simulink model "Simulator"  (R2024b)
settings: Solver=FixedStepAuto  StartTime=0.0  StopTime=Parameters.Simulink.sim_time_s  FixedStep=Parameters.Simulink.time_step_s  RelTol=1e-6
undefined symbols (not defined in the file): att_0, data, flight_mode, FLIGHT_MODE, id, joystick, Parameters, res, timestamp, traj_opt, wait_time_s
libraries: dspsigops x3, simulink x2, eeGeneralControl x2, px4uORBlib x2, vrlib x1, simulink_extras x1, aerolibanimutils x1, sharedtransform x1
(part 2 of 2)

== system Simulator/Guidance/Subsystem2/minimum_snap/Subsystem/re-solve trajectory/Enabled Subsystem1/Subsystem3 ==
  States : Inport
  Bus Selector2 : BusSelector  OutputSignals=a_e,omega_dot
  Discrete Derivative : simulink/Discrete/Discrete Derivative  gainval=1.0  ICPrevScaledInput=0.0  OutMin=[]  OutMax=[]  OutDataType=fixdt(1, 16)  OutScaling=2^-10  DoSatur=off
  Discrete Derivative1 : simulink/Discrete/Discrete Derivative  gainval=1.0  ICPrevScaledInput=0.0  OutMin=[]  OutMax=[]  OutDataType=fixdt(1, 16)  OutScaling=2^-10  DoSatur=off
  Low-Pass Filter (Discrete or Continuous) : eeGeneralControl/Low-Pass Filter (Discrete or Continuous)  K=1  T=0.1  B=inf  A=-inf  init_option=Inherited from block input  x0=0  Ts=-1
  Low-Pass Filter (Discrete or Continuous)1 : eeGeneralControl/Low-Pass Filter (Discrete or Continuous)  K=1  T=0.1  B=inf  A=-inf  init_option=Inherited from block input  x0=0  Ts=-1
  Mux : Mux  Inputs=2
  Reshape : Reshape
  Reshape1 : Reshape
  Selector : Selector  InputPortWidth=3  IndexOptions=Index vector (dialog)  Indices=[3]  OutputSizes=1
  state_vec_jerk : Outport
  state_vec_snap : Outport  Port=2
  wires:
  Bus Selector2/1 -> Reshape/1  "<a_e>"
  Reshape1/1 -> Mux/2
  Selector/1 -> Reshape1/1
  Bus Selector2/2 -> Selector/1  "<omega_dot>"
  Reshape/1 -> Mux/1
  States/1 -> Bus Selector2/1
  Mux/1 -> Discrete Derivative/1
  Discrete Derivative/1 -> Low-Pass Filter (Discrete or Continuous)/1
  Low-Pass Filter (Discrete or Continuous)/1 -> Discrete Derivative1/1, state_vec_jerk/1
  Discrete Derivative1/1 -> Low-Pass Filter (Discrete or Continuous)1/1
  Low-Pass Filter (Discrete or Continuous)1/1 -> state_vec_snap/1

== system Simulator/Inbound Data/Subsystem4/Subsystem/Subsystem1/Sliders/Subsystem2/If Action Subsystem ==
  Action Port : ActionPort
  Clock : Clock
  Constant : Constant  Value=flight_mode.autonomous
  Constant1 : Constant  Value=flight_mode.position_hold
  Constant2 : Constant  Value=wait_time_s
  GreaterThan : RelationalOperator  Operator=<  OutDataTypeStr=boolean  RndMeth=Simplest  InputSameDT=off
  Multiport Switch1 : MultiPortSwitch  DataPortOrder=Zero-based contiguous  Inputs=2  DiagnosticForDefault=None  zeroidx=on  SaturateOnIntegerOverflow=off  InputSameDT=off
  Out1 : Outport
  wires:
  Constant2/1 -> GreaterThan/2
  Constant1/1 -> Multiport Switch1/3
  GreaterThan/1 -> Multiport Switch1/1
  Constant/1 -> Multiport Switch1/2
  Multiport Switch1/1 -> Out1/1
  Clock/1 -> GreaterThan/1

== system Simulator/Inbound Data/Subsystem4/Subsystem/Subsystem1/Sliders/Subsystem2/If Action Subsystem1 ==
  In1 : Inport
  Action Port : ActionPort
  Out1 : Outport
  wires:
  In1/1 -> Out1/1

== matlab function Simulator/Inbound Data/Subsystem3/Trajectory Solution/Call solver/Enabled Subsystem/MATLAB Function ==
  settings: updateMethod=DISCRETE  sampleTime=Parameters.Simulink.time_step_s
  data: trajectory_id input size=1; T_new output size=[1,100]; pp_new output size=[99,10,4]; n_dim_new output size=1; n_dim_ids_new output size=[4,1]; N_segments_new output size=1
function [T_new, pp_new, n_dim_new, n_dim_ids_new, N_segments_new]...
    = traj_solver(trajectory_id)
[wpts, Tf] = trajectory_manager.get_traj(trajectory_ID(trajectory_id));

opt_time_allocation_fl = false;
ShowDetails = false;

[T_new, pp_new, n_dim_new, n_dim_ids_new, N_segments_new, offset_new, Cost, ExitFlag, Iterations] = solver_codegen(wpts, Tf, ...
    opt_time_allocation_fl, ShowDetails);
end

== matlab function Simulator/Guidance/Subsystem2/minimum_snap/Subsystem/use static solution/MATLAB Function ==
  settings: updateMethod=DISCRETE  sampleTime=Parameters.Simulink.time_step_s
  data: t input size=1; p output size=[3,1]; v output size=[3,1]; a output size=[3,1]; jerk output size=[3,1]; T input double [0..]; coefs input double; snap output size=[3,1]; psi output size=1; psi_dot output size=1; psi_ddot output size=1; finished_traj output size=1; n_dim input; n_dim_src input; n_dim_ids input; n_int input; waypoints_offset input; gen_FF_fl input
function [p, v, a, jerk, snap, psi, psi_dot, psi_ddot, finished_traj] = eval_traj(...
    t,T,coefs,n_dim,n_dim_src, n_dim_ids, n_int, waypoints_offset, gen_FF_fl)

if isempty(T)
    finished_traj = true;
    p           = zeros(3,1);
    
    v           = zeros(3,1);
    p(:)        = waypoints_offset(1:3);
    a           = zeros(3,1);
    jerk        = zeros(3,1);
    snap        = zeros(3,1);
    psi         = waypoints_offset(4);
    psi_dot     = 0;
    psi_ddot    = 0;
else
    TU_input_factor = 10 / T(end);
    DU_input_factor = 1;
    
    if gen_FF_fl
        [p, v, a, jerk, snap, psi, psi_dot, psi_ddot, finished_traj] = eval_traj(...
            t,T,coefs,n_dim,n_dim_src, n_dim_ids, n_int, waypoints_offset, DU_input_factor, TU_input_factor);
    else
        [p, ~, ~, ~, ~, psi, ~, ~, finished_traj] = eval_traj(...
        t,T,coefs,n_dim,n_dim_src, n_dim_ids, n_int, waypoints_offset, DU_input_factor, TU_input_factor);
        v           = zeros(3,1);
        a           = zeros(3,1);
        jerk        = zeros(3,1);
        snap        = zeros(3,1);
        psi_dot     = 0;
        psi_ddot    = 0;
    end
end
end

== matlab function Simulator/Guidance/Subsystem2/Step input/MATLAB Function ==
  data: t input; pos output; yaw output; pos input; yaw input; completed output
function [pos, yaw, completed] = fcn(t, pos, yaw)
% pos = zeros(3,1);
% vel = zeros(3,1);
% att = zeros(3,1);
% att_rate = zeros(3,1);
completed = 0;

if t > 23
    completed = 1;
elseif t > 12
    pos(1) = pos(1) + 2;
    pos(2) = pos(2);
    pos(3) = pos(3) + 1;
elseif t > 6
    pos(1) = pos(1) + 2;
    pos(2) = pos(2);
else
    pos(1) = pos(1) + 1;
    pos(2) = pos(2) + 1;
end
end

== matlab function Simulator/Guidance/Subsystem2/minimum_snap/Subsystem/re-solve trajectory/Enabled Subsystem1/MATLAB Function ==
  settings: updateMethod=DISCRETE  sampleTime=Parameters.Simulink.time_step_s
  data: p output size=[3,1]; v output size=[3,1]; a output size=[3,1]; jerk output size=[3,1]; snap output size=[3,1]; psi output size=1; psi_dot output size=1; psi_ddot output size=1; finished_traj output size=1; guidance_active input; trajectory_id input size=1; time_since_start_of_traj_glob input size=1; update_dt input; T_glob input; pp_glob input; n_dim_glob input; n_dim_src_glob input; n_dim_ids_glob input; N_segments_glob input; state_0_glob input; time_since_start_of_traj output size=1; T output size=[1,100]; pp output size=[99,10,4]; n_dim output; n_dim_src output size=1; n_dim_ids output size=[4,1]; N_segments output size=1; state_0 output; state_vec input; detection_range input; waypoint_keepout_range input; collision_check_tol input; wpts output size=[4,100]
function [p, v, a, jerk, snap, psi, psi_dot, psi_ddot, finished_traj,...
            time_since_start_of_traj, T, pp, n_dim, n_dim_src, n_dim_ids, N_segments, state_0, wpts]...
            = update_and_eval_traj(guidance_active, trajectory_id, ...
            time_since_start_of_traj_glob, update_dt, ...
            T_glob, pp_glob, n_dim_glob, n_dim_src_glob, n_dim_ids_glob, N_segments_glob, ...
            state_0_glob, ...
            state_vec,... %, state_vec_vel, state_vec_acc, state_vec_jerk, state_vec_snap)
            detection_range, waypoint_keepout_range, collision_check_tol) 

persistent p_prev_ v_prev_ a_prev_ jerk_prev_ snap_prev_ psi_prev_ psi_dot_prev_ psi_ddot_prev_;

if (isempty(p_prev_) || isempty(v_prev_) || isempty(a_prev_) || isempty(jerk_prev_) || isempty(snap_prev_) || isempty(psi_prev_) ...
            || isempty(psi_dot_prev_) || isempty(psi_ddot_prev_))
    p_prev_ = zeros(3,1);
    p_prev_(:) = state_0_glob(1:3);
    v_prev_ = zeros(3,1);
    a_prev_ = zeros(3,1);
    jerk_prev_ = zeros(3,1);
    snap_prev_ = zeros(3,1);
    % psi_prev_ = 0;
    psi_prev_ = state_0_glob(4);
    psi_dot_prev_ = 0;
    psi_ddot_prev_ = 0;
end

[T, pp, n_dim, n_dim_src, n_dim_ids, N_segments, ...
    time_since_start_of_traj, state_0, wpts]...
            = traj_solver_...
            (guidance_active, trajectory_id, ...
            time_since_start_of_traj_glob, update_dt, ...
            T_glob, pp_glob, n_dim_glob, n_dim_src_glob, n_dim_ids_glob, N_segments_glob, ...
            state_0_glob, ...
            state_vec, ...% state_vec_vel, state_vec_acc, state_vec_jerk, state_vec_snap,...
            p_prev_, v_prev_, a_prev_, jerk_prev_, snap_prev_, psi_prev_, psi_dot_prev_, psi_ddot_prev_,...
            detection_range, waypoint_keepout_range, collision_check_tol);


[p, v, a, jerk, snap, psi, psi_dot, psi_ddot, finished_traj] = eval_traj_(...
    time_since_start_of_traj, T, pp, n_dim, n_dim_src, n_dim_ids, N_segments, state_0);


p_prev_(:) = p(1:3);
v_prev_(:) = v(1:3);
a_prev_(:) = a(1:3);
jerk_prev_(:) = jerk(1:3);
snap_prev_(:) = snap(1:3);
psi_prev_ = psi(1);
psi_dot_prev_ = psi_dot(1);
psi_ddot_prev_ = psi_ddot(1);

end


function [p, v, a, jerk, snap, psi, psi_dot, psi_ddot, finished_traj] = eval_traj_(...
    t,T,coefs,n_dim,n_dim_src, n_dim_ids, n_int, waypoints_offset)

    if isempty(T)
        finished_traj = true;
        p           = zeros(3,1);        
        v           = zeros(3,1);
        p(:)        = waypoints_offset(1:3);
        a           = zeros(3,1);
        jerk        = zeros(3,1);
        snap        = zeros(3,1);
        psi         = waypoints_offset(4);
        psi_dot     = 0;
        psi_ddot    = 0;
    else
        TU_input_factor = 10 / T(end);
        DU_input_factor = 1;
        
        [p, v, a, jerk, snap, psi, psi_dot, psi_ddot, finished_traj] = eval_traj(...
            t,T,coefs,n_dim,n_dim_src, n_dim_ids, n_int, waypoints_offset, DU_input_factor, TU_input_factor);
    end
end






function [T, pp, n_dim, n_dim_src, n_dim_ids, N_segments, ...
    time_since_start_of_traj, state_0, wpts]...
            = traj_solver_...
            (guidance_active, trajectory_id, ...
            time_since_start_of_traj_glob, update_dt, ...
            T_glob, pp_glob, n_dim_glob, n_dim_src_glob, n_dim_ids_glob, N_segments_glob, ...
            state_0_glob, ...
            state_vec, ...% state_vec_vel, state_vec_acc, state_vec_jerk, state_vec_snap,...
            p_prev, v_prev, a_prev, jerk_prev, snap_prev, psi_prev, psi_dot_prev, psi_ddot_prev,...
            detection_range, waypoint_keepout_range, collision_check_tol)
    
    %initialization:
    persistent T_  pp_ n_dim_ n_dim_src_ n_dim_ids_ N_segments_ time_since_start_of_traj_ status_int_ state_0_ wpts_ obstcl_;
    coder.varsize('T_',[1 inf], [0 1]);
    coder.varsize('pp_',[inf 10 inf]);
    coder.varsize('n_dim_ids_',[4 1], [1 0]);
    coder.varsize('wpts_',[4 inf], [1 1]);
    coder.varsize('obstcl_',[1 inf], [1 1]);
    
    if (isempty(obstcl_))
        [~, obstcl_] = trajectory_manager.get_traj(trajectory_ID(trajectory_id));
    end

    if (isempty(T_) || isempty(pp_) || isempty(n_dim_) || isempty(n_dim_src_) || isempty(n_dim_ids_) || isempty(N_segments_) ...
            || isempty(time_since_start_of_traj_) || isempty(status_int_) || isempty(state_0_)) || isempty(wpts_) ...
        T_ = T_glob(:)';
        pp_ = pp_glob;
        n_dim_ = n_dim_glob;
        n_dim_src_ = n_dim_src_glob;
        n_dim_ids_ = n_dim_ids_glob;
        N_segments_ = N_segments_glob;
        time_since_start_of_traj_ = time_since_start_of_traj_glob;
        status_int_ = 0;
        state_0_ = state_0_glob;
        [wpts_] = trajectory_manager.get_traj(trajectory_ID(trajectory_id));


        T = T_;
        pp = pp_;
        n_dim = n_dim_;
        n_dim_src = n_dim_src_;
        n_dim_ids = n_dim_ids_;
        N_segments = N_segments_;
        time_since_start_of_traj = time_since_start_of_traj_;
        state_0 = state_0_;
        wpts = wpts_;
        return;
    end

    % state_0 = zeros(4,1); %x, y, z, yaw

    if status_int_ == 2 && ~guidance_active
        status_int_ = 1;
    end

    switch status_int_
        case 2 % this time we will actually re-solve the trajectory            
            % the routine is after the switch-case 
            % (don't return here)

        case 1 % check timing and request to solve a trajectory (keep old result)
            % trajectory_update_dt_s = .1;

            % if rem(time_since_start_of_traj_glob,trajectory_update_dt_s) == 0 %time to update (time-based)
            for i = 1:length(obstcl_)
                if obstcl_{i}.check_if_obs_is_interior(state_vec(1:3), detection_range)
                    obstcl_{i}.is_visible = true;
                    if (~obstcl_{i}.was_processed)
                        if time_since_start_of_traj_glob > 0.0 && time_since_start_of_traj_ < T_(N_segments_+1)
                            disp(time_since_start_of_traj_glob)
                            status_int_ = 2;
                        end
                    end
                else
                    obstcl_{i}.is_visible = false;
                    % obstcl_{i}.was_processed = false;
                end
            end


            T = T_;
            pp = pp_;
            n_dim = n_dim_;
            n_dim_src = n_dim_src_;
            n_dim_ids = n_dim_ids_;
            N_segments = N_segments_;
            time_since_start_of_traj_ = (time_since_start_of_traj_ + update_dt);
            time_since_start_of_traj = time_since_start_of_traj_;
            state_0 = state_0_;
            wpts = wpts_;
            return;
            
            
        otherwise % don't solve anything just pass global solution and update status
            T_ = T_glob(:)';
            pp_ = pp_glob;
            n_dim_ = n_dim_glob;
            n_dim_src_ = n_dim_src_glob;
            n_dim_ids_ = n_dim_ids_glob;
            N_segments_ = N_segments_glob;
            time_since_start_of_traj_ = time_since_start_of_traj_glob;
            state_0_ = state_0_glob;
    
    
            T = T_;
            pp = pp_;
            n_dim = n_dim_;
            n_dim_src = n_dim_src_;
            n_dim_ids = n_dim_ids_;
            N_segments = N_segments_;
            time_since_start_of_traj = time_since_start_of_traj_;
            state_0 = state_0_;
            wpts = wpts_;
            
            if guidance_active && time_since_start_of_traj_glob > 0.0 && ~isempty(T_) && time_since_start_of_traj_glob < T_(N_segments_+1)
                %trajectory guidance is active, start checking stuff
                status_int_ = 1; 
            end
            return;
    end
    
    % use state:
    % state_0__ = state_vec(1:4); % we will output a new intial state
    
    % alternatively we can use the last setpoint:
    state_0__ = [p_prev(1:3); psi_prev(1)]; % we will output a new intial state

    %we want to remove the completed waypoints:
    completed_segments = time_since_start_of_traj_ + update_dt >= T_;
    N_remove_segments = nnz(completed_segments) - 1;

    N_segments_traj = size(wpts_,2) - 1;
    wpts_mod_ = wpts_(:,N_remove_segments+1:N_segments_traj+1); %for now, we make a local copy (we may discard this later)
    
    %let's evaluate the trajectory ahead of us to check for the collisions
    % first, we need to make sure we keep the "old" parameters needed for
    % trajectory evaluation (mainly time) 
    Tf =T_(N_segments_+1); % total flight time (for old trajectory)
    T_mod_ = T_(N_remove_segments+1:N_segments_traj+1) - time_since_start_of_traj_; %this is cropped time vector
    T_mod_(1) = 0; % make sure new time vector starts at 0
    eval_time_ahead__ = time_since_start_of_traj_+update_dt:0.1:T_(N_segments_+1); %evaluation has to be relative to the old time vector
    TU_input_factor__ = 10 / Tf; %time scaling (old)
    p_look_ahead__ = TrajectoryOptimizer.common.eval_pp(...
                eval_time_ahead__,...
                0,...
                pp_, ...
                T_, ...
                n_dim_,...
                n_dim_src_, ...
                n_dim_ids_, ...
                N_segments_, ...
                state_0_, ...
                1, ...
                TU_input_factor__); %we do this once and use to check all obstacles
    eval_time_ahead__ = eval_time_ahead__-time_since_start_of_traj_; %offset by the flown time 

    requires_trajectory_update = false; %we mat actually have no collision with any of the obstacles, so don't update just because... 
    
    for i = 1:length(obstcl_) %checking every obstacle
        if obstcl_{i}.is_visible && ~obstcl_{i}.was_processed %only visible and those that have not been processed yet
            [is_interior__, n_new_wpts__, new_wpts__, new_wpt_T__] = obstcl_{i}.check_traj(eval_time_ahead__, p_look_ahead__(1:3,:), collision_check_tol, waypoint_keepout_range);
            if nnz(is_interior__) > 0 % only if any of the points are inside the obstacles
                [wpts_mod_, T_mod_] = obstcl_{i}.insert_new_wpts(new_wpt_T__, n_new_wpts__, new_wpts__, wpts_mod_, T_mod_, collision_check_tol); %updates waypoints and time vector
                % obstcl_{i}.was_processed = true;
                requires_trajectory_update = true;
                for ii = 1:length(obstcl_)
                    if obstcl_{ii}.is_visible
                        obstcl_{ii}.was_processed = false;
                    end
                end
            end
        end
    end

    if requires_trajectory_update %only if needed
        %here we will compute a new trajectory based on the updated
        %waypoints and time vector
        T_ = T_mod_;
        wpts_ = wpts_mod_;
    
        Tf = T_(end);    
        wpts_(:,1) = state_0__(1:4);   
    
        opt_time_allocation_fl = false;
        ShowDetails = false;        
        timeWt = 0;
        
        scaling = 10;
        
        minSegmentTime = 0.1*diff(T_);
        maxSegmentTime = Tf;
        
        % wptFun = @(t) bcs_fun1__(t, wpts);
        wptFun = @(t) bcs_fun2__(t, wpts_, v_prev, a_prev, jerk_prev, snap_prev, psi_dot_prev, psi_ddot_prev);
        % wptFun = @(t)bcs_fun3__(t, wpts, state_vec_vel, state_vec_acc, state_vec_jerk, state_vec_snap);
        
        sol = TrajectoryOptimizer.solver_mexfriendy( ...
            T_,...
            opt_time_allocation_fl,...
            ShowDetails, ...
            wptFun, ...
            [], ...
            minSegmentTime, ...
            maxSegmentTime, ...
            timeWt, ...
            scaling / Tf);
        
        % stats = sol.get_stats;
        minsnap_set = sol.get_res;
    
        % ExitFlag = stats.ExitFlag;
        % Iterations = stats.Iterations;
        % Cost = stats.J;
    
        pp = minsnap_set.pp;
        T = minsnap_set.T;
        n_dim = minsnap_set.n_dim;
        n_dim_src = minsnap_set.n_dim_src;
        n_dim_ids = minsnap_set.n_dim_ids;
        N_segments = minsnap_set.N_segments;
        state_0 = state_0__;
        time_since_start_of_traj = update_dt;
    
        status_int_ = 1; %return back to 1 by default
        T_ = T;
        pp_ = pp;
        n_dim_ = n_dim;
        n_dim_src_ = n_dim_src;
        n_dim_ids_ = n_dim_ids;
        N_segments_ = N_segments;
        time_since_start_of_traj_ = time_since_start_of_traj;
        state_0_ = state_0__;   
        wpts = wpts_;

    else % we will check again on the next iteration
        for ii = 1:length(obstcl_)
            if obstcl_{ii}.is_visible && ~obstcl_{ii}.was_processed
                obstcl_{ii}.was_processed = true;
            end
        end
        T = T_;
        pp = pp_;
        n_dim = n_dim_;
        n_dim_src = n_dim_src_;
        n_dim_ids = n_dim_ids_;
        N_segments = N_segments_;
        time_since_start_of_traj_ = (time_since_start_of_traj_ + update_dt);
        time_since_start_of_traj = time_since_start_of_traj_;
        state_0 = state_0_;
        status_int_ = 1; %return back to 1 by default
        wpts = wpts_;
    end

    function [wpts, extra_bcs] = bcs_fun1__(~, wpts)
        extra_bcs = {};
    end

    function [wpts, extra_bcs] = bcs_fun2__(~, wpts, v, a, jerk, snap, psi_dot, psi_ddot)
        n_dt = 4;
        extra_bcs = cell(1,n_dt);
        [n_dims, n_wpts] = size(wpts);
        % extra_bcs(:) = {NaN(n_dims, n_wpts)};
        for i_dt = 1:n_dt
            extra_bcs{i_dt} = NaN(n_dims,n_wpts);
        end
        extra_bcs{1}(1:3,1) = v(:);
        extra_bcs{2}(1:3,1) = a(:);
        extra_bcs{3}(1:3,1) = jerk(:);
        extra_bcs{4}(1:3,1) = snap(:);
        extra_bcs{1}(4,1) = psi_dot;
        extra_bcs{2}(4,1) = psi_ddot;
        for i_dt = 1:n_dt
            for i_dim = 1:n_dims
                extra_bcs{i_dt}(i_dim,n_wpts) = 0;
            end
        end
    end

    function [wpts, extra_bcs] = bcs_fun3__(~, wpts, wpts_v, wpts_a, wpts_jerk, wpts_snap)
        n_dt = 4;
        extra_bcs = cell(1,n_dt);
        [n_dims, n_wpts] = size(wpts);
        % extra_bcs(:) = {NaN(n_dims, n_wpts)};
        for i_dt = 1:n_dt
            extra_bcs{i_dt} = NaN(n_dims,n_wpts);
        end
        extra_bcs{1}(1:4,1) = wpts_v(:);
        extra_bcs{2}(1:4,1) = wpts_a(:);
        extra_bcs{3}(1:4,1) = wpts_jerk(:);
        extra_bcs{4}(1:4,1) = wpts_snap(:);
        for i_dt = 1:n_dt
            for i_dim = 1:n_dims
                extra_bcs{i_dt}(i_dim,n_wpts) = 0;
            end
        end
    end
end

== matlab function Simulator/Subsystem/Controller with PX4 IO/GUIDANCE_MSG_MAP/MATLAB Function ==
  data: pos input; GUIDANCE_DATA_MSG output; vel input; acc input; jerk input; snap input; yaw input; yaw_rate input; yaw_acc input; yaw_jerk input; yaw_snap input; completed input
function GUIDANCE_DATA_MSG  = translation_guidance2msg(pos, vel, acc, jerk, snap,...
    yaw, yaw_rate, yaw_acc, yaw_jerk, yaw_snap, completed)

MAX_SIZE = 58;
GUIDANCE_DATA_MSG = zeros(1,MAX_SIZE);
N_DOFS = 4;
pos_ = [pos(:);yaw(1)];
vel_ = [vel(:);yaw_rate(1)];
acc_ = [acc(:);yaw_acc(1)];
jerk_ = [jerk(:);yaw_jerk(1)];
snap_ = [snap(:);yaw_snap(1)];

ind = 0;
ind = ind+1;
GUIDANCE_DATA_MSG(ind) = double(completed(1));

for i = 1:N_DOFS
    ind = ind + 1;
    GUIDANCE_DATA_MSG(ind) = pos_(i);
end
for i = 1:N_DOFS
    ind = ind + 1;
    GUIDANCE_DATA_MSG(ind) = vel_(i);
end
for i = 1:N_DOFS
    ind = ind + 1;
    GUIDANCE_DATA_MSG(ind) = acc_(i);
end
for i = 1:N_DOFS
    ind = ind + 1;
    GUIDANCE_DATA_MSG(ind) = jerk_(i);
end
for i = 1:N_DOFS
    ind = ind + 1;
    GUIDANCE_DATA_MSG(ind) = snap_(i);
end

end

== matlab function Simulator/Inbound Data/Subsystem4/Subsystem/Subsystem1/Joytick/MATLAB Function ==
  data: sticks input; roll_stick output; buttons input; n input; min input; max input; pitch_stick output; yaw_stick output; throttle_stick output; vals input; FLIGHT_MODE output
function [roll_stick, pitch_stick, yaw_stick, throttle_stick, FLIGHT_MODE] = fcn(sticks, buttons, n, min, max, vals)
joystick.sticks.raw = sticks;
joystick.buttons.raw = buttons;
joystick.sticks.n = n;
joystick.sticks.cal.min = min;
joystick.sticks.cal.max = max;
joystick.sticks.cal.vals = vals;

ROLL_STICK = 1;
PITCH_STICK = 2;
THROTTLE_STICK = 3;
YAW_STICK = 5;
AUX1_STICK = 4;

StickMap = [...
    ROLL_STICK
    PITCH_STICK
    YAW_STICK
    THROTTLE_STICK
    AUX1_STICK];

ROLL_STICK_POL = 1;
PITCH_STICK_POL = -1;
THROTTLE_STICK_POL = -1;
YAW_STICK_POL = 1;
AUX1_STICK_POL = 1;

StickPol = [...
    ROLL_STICK_POL
    PITCH_STICK_POL
    YAW_STICK_POL
    THROTTLE_STICK_POL
    AUX1_STICK_POL];

% tol = 1E-12;
deadzone_RPY = 0.05; %sticks are not perfectly centered 
deadzone_Z = 0.05;
joystick = lib.joystick.apply_cal(joystick);
mapped_sticks = joystick.sticks.cal.vals(StickMap);
mapped_sticks = mapped_sticks(:).*StickPol(:);
roll_stick = lib.math.apply_deadzone(mapped_sticks(1),deadzone_RPY,0);
pitch_stick = lib.math.apply_deadzone(mapped_sticks(2),deadzone_RPY,0);
yaw_stick = lib.math.apply_deadzone(mapped_sticks(3),deadzone_RPY,0);
throttle_stick = lib.math.apply_deadzone(mapped_sticks(4),deadzone_Z,0);

button_case = 0;
flight_mode_buttons = buttons(4:5);
if flight_mode_buttons(1) == 0 && flight_mode_buttons(2) == 0
    button_case = 0;
elseif flight_mode_buttons(1) == 1
    button_case = 1;
elseif flight_mode_buttons(2) == 1
    button_case = 2;
end


switch button_case
    case 2
        FLIGHT_MODE = flight_mode.autonomous;
    case 1
        FLIGHT_MODE = flight_mode.attitude_control;
        % FLIGHT_MODE = flight_mode.position_control;
    case 0
        % FLIGHT_MODE = flight_mode.attitude_control;
        FLIGHT_MODE = flight_mode.position_control;
    otherwise 
        FLIGHT_MODE = flight_mode.position_hold;
end

end

== matlab function Simulator/Guidance/Subsystem1/MATLAB Function ==
  data: mode_request input Enum: flight_mode size=1; current_mode output; current_mode input Enum: flight_mode size=1; timer input; wait_time input; reset output; timer output
function [current_mode, reset, timer] = fcn(mode_request, current_mode, timer, wait_time)
reset = false;

if mode_request == current_mode
    timer = 0;
    return
end

switch mode_request
    case flight_mode.autonomous
        switch current_mode
            case flight_mode.position_hold
                if timer > wait_time
                    current_mode = flight_mode.autonomous;                    
                    timer = 0;
                else
                    timer = timer + 1;
                end
                return;
            otherwise
                current_mode = flight_mode.position_hold;
                reset = true;
                timer = 0;
                return;                

        end
    case flight_mode.position_hold
        switch current_mode
            case flight_mode.attitude_control
                current_mode = flight_mode.position_hold;
                reset = true;
                timer = 0;
                return;
            case flight_mode.autonomous
                current_mode = flight_mode.position_hold;
                reset = true;
                timer = 0;
            otherwise
                current_mode = mode_request;
                timer = 0;
                return;                

        end
    case flight_mode.position_control
        switch current_mode
            case flight_mode.attitude_control
                current_mode = flight_mode.position_control;
                reset = true;
                timer = 0;
                return;
            case flight_mode.autonomous
                current_mode = flight_mode.position_control;
                reset = true;
                timer = 0;
            otherwise
                current_mode = mode_request;
                timer = 0;
                return;                

        end
    otherwise
        current_mode = mode_request;
        timer = 0;
        return;
end

end
